simulink model "phase_lead_control_open_loop_system"  (R2020b)
settings: Solver=VariableStepAuto  StartTime=0.0  StopTime=200  RelTol=1e-3
values from neighbouring files (symbols this model uses):
  COMMANDED_TORQUE_SATURATION = 0.05    [Workshop_MATLAB.m]
  COUPLING_COEFFICIENT = 0.5736    [Workshop_MATLAB.m]
  ESTIMATOR_TRANSFER_FUNCTION_DENOMINATOR = [ESTIMATOR_TIME_CONSTANT 1]    [Workshop_MATLAB.m]
  ESTIMATOR_TRANSFER_FUNCTION_NUMERATOR = [1 0]    [Workshop_MATLAB.m]
  FLEXIBLE_MODE_DAMPING_RATIO = 0.00495    [Workshop_MATLAB.m]
  FLEXIBLE_MODE_FREQUENCY = 2.6268    [Workshop_MATLAB.m]
  INITIAL_CONDITION_ON_STATE = 0.0001    [Workshop_MATLAB.m]
  REACTION_WHEEL_DYNAMICS_DENOMINATOR = [1 2.400 0.763]    [Workshop_MATLAB.m]
  REACTION_WHEEL_DYNAMICS_NUMERATOR = REACTION_WHEEL_INERTIA*[1.214 0.763 0]    [Workshop_MATLAB.m]
  REACTION_WHEEL_INERTIA = 0.0004    [Workshop_MATLAB.m]
  REACTION_WHEEL_VELOCITY_SATURATION = 2800*2*pi/60    (= 293.215314335)    [Workshop_MATLAB.m]
  SATELLITE_INERTIA = 31.38    [Workshop_MATLAB.m]
settings Model: Creator=WLCG  LastModifiedBy=WLCG

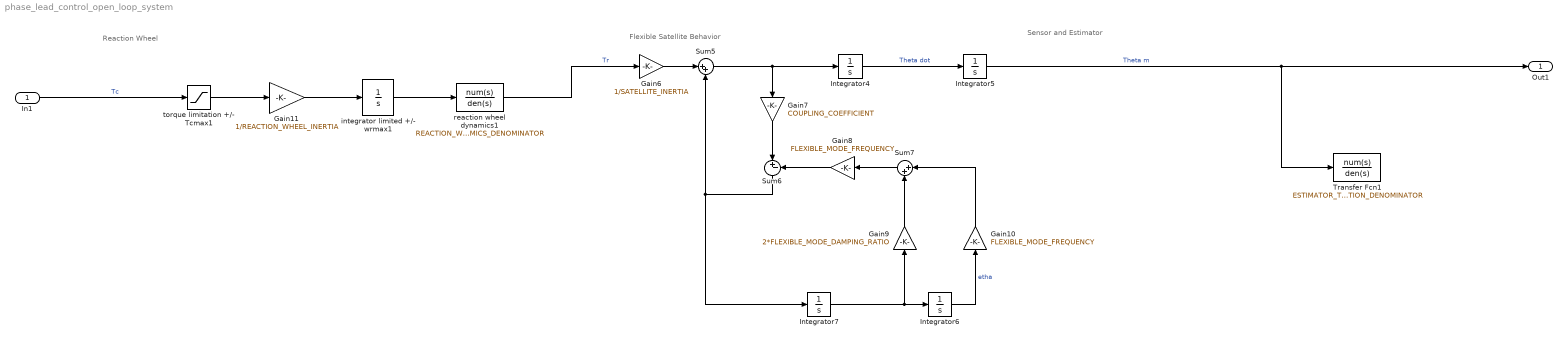
== system phase_lead_control_open_loop_system ==
  note: Sensor and Estimator
  note: Flexible Satellite Behavior
  note: Reaction Wheel
  In1 : Inport
  Gain10 : Gain  Gain=FLEXIBLE_MODE_FREQUENCY
  Gain11 : Gain  Gain=1/REACTION_WHEEL_INERTIA
  Gain6 : Gain  Gain=1/SATELLITE_INERTIA
  Gain7 : Gain  Gain=COUPLING_COEFFICIENT
  Gain8 : Gain  Gain=FLEXIBLE_MODE_FREQUENCY
  Gain9 : Gain  Gain=2*FLEXIBLE_MODE_DAMPING_RATIO
  Integrator4 : Integrator
  Integrator5 : Integrator
  Integrator6 : Integrator  InitialCondition=INITIAL_CONDITION_ON_STATE
  Integrator7 : Integrator
  Sum5 : Sum  Inputs=|++
  Sum6 : Sum  Inputs=|+-
  Sum7 : Sum  Inputs=|++
  Transfer Fcn1 : TransferFcn  Numerator=ESTIMATOR_TRANSFER_FUNCTION_NUMERATOR  Denominator=ESTIMATOR_TRANSFER_FUNCTION_DENOMINATOR
  integrator limited +/- wrmax1 : Integrator  LimitOutput=on  UpperSaturationLimit=REACTION_WHEEL_VELOCITY_SATURATION  LowerSaturationLimit=-REACTION_WHEEL_VELOCITY_SATURATION
  reaction wheel dynamics1 : TransferFcn  Numerator=REACTION_WHEEL_DYNAMICS_NUMERATOR  Denominator=REACTION_WHEEL_DYNAMICS_DENOMINATOR
  torque limitation +/- Tcmax1 : Saturate  UpperLimit=COMMANDED_TORQUE_SATURATION  LowerLimit=-COMMANDED_TORQUE_SATURATION
  Out1 : Outport
  wires:
  In1/1 -> torque limitation +/- Tcmax1/1  "Tc"
  Gain7/1 -> Sum6/1
  Gain9/1 -> Sum7/2
  Sum7/1 -> Gain8/1
  Integrator5/1 -> Transfer Fcn1/1, Out1/1  "Theta m"
  Gain10/1 -> Sum7/1
  reaction wheel dynamics1/1 -> Gain6/1  "Tr"
  Gain8/1 -> Sum6/2
  Integrator4/1 -> Integrator5/1  "Theta dot"
  torque limitation +/- Tcmax1/1 -> Gain11/1
  Gain6/1 -> Sum5/1
  Gain11/1 -> integrator limited +/- wrmax1/1
  Sum5/1 -> Gain7/1, Integrator4/1
  Integrator6/1 -> Gain10/1  "etha"
  Integrator7/1 -> Integrator6/1, Gain9/1
  integrator limited +/- wrmax1/1 -> reaction wheel dynamics1/1
  Sum6/1 -> Sum5/2, Integrator7/1
